simulink model "verify_alfa_window_out_mdl"  (R2016b)
settings: Solver=VariableStepDiscrete  StartTime=12*3600  StopTime=20+12*3600  MaxStep=1  RelTol=1e-3  EnableMultiTasking=on
libraries: carnot x2, simulink x1
settings Model: Creator=drhf  LastModifiedBy=srrt
settings DataIOCC: SaveFormat=Array  SignalLoggingSaveFormat=ModelDataLogs
settings OptimizationCC: ExpressionDepthLimit=2147483647  LifeSpan=inf
settings DebuggingCC: UnderspecifiedInitializationDetection=Classic  MergeDetectMultiDrivingBlocksExec=none  SolverPrmCheckMsg=warning  FcnCallInpInsideContextMsg=warning  StateNameClashWarn=warning  SFUnexpectedBacktrackingDiag=warning  SFNoUnconditionalDefaultTransitionDiag=warning  SFExecutionAtInitializationDiag=none
settings HardwareCC: ProdBitPerPointer=32  ProdBitPerSizeT=32  ProdBitPerPtrDiffT=32  ProdLargestAtomicFloat=None  ProdIntDivRoundTo=Undefined  ProdEndianess=Unspecified  ProdWordSize=32  ProdHWDeviceType=32-bit Generic
settings ModelReferenceCC: PropagateSignalLabelsOutOfModel=off
settings GRTTargetCC: TargetLangStandard=C89/C90 (ANSI)  GeneratePreprocessorConditionals=Disable all  CombineOutputUpdateFcns=off  GRTInterface=on
settings ConfigComp: CovMetricSettings=dw  CovHtmlReporting=on  CovSaveCumulativeToWorkspaceVar=on  CovSaveSingleToWorkspaceVar=on  CovExternalEMLEnable=off

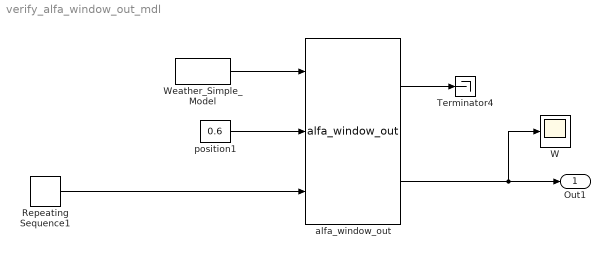
== system verify_alfa_window_out_mdl ==
  Repeating Sequence1 : simulink/Sources/Repeating Sequence  rep_seq_t=[0 10]  rep_seq_y=[10 30]
  Terminator4 : Terminator
  W : Scope
  Weather_Simple_Model : carnot/Weather/Weather_Simple_Model  lat=60  Ibn=900  Idg=100  tamb=5  deltaTsky=-6  rh=50  precip="10e-3/24/3600           % 10 mm in 24 h"  cloud=0.125  p=1013e2  vw=1  wdir=270
  alfa_window_out : carnot/Load/Houses/heat_transfer/alfa_window_out  pos=0  absorption_out=0.01  emission_out=0.87  frame=0.1
  position1 : Constant  Value=0.6
  Out1 : Outport
  wires:
  Repeating Sequence1/1 -> alfa_window_out/3
  Weather_Simple_Model/1 -> alfa_window_out/1
  position1/1 -> alfa_window_out/2
  alfa_window_out/2 -> W/1, Out1/1
  alfa_window_out/1 -> Terminator4/1
